simulink model "lab61"  (R2023b)
settings: Solver=VariableStepAuto  StartTime=0.0  StopTime=100  RelTol=1e-3
model workspace (MAT data in the model file):
  a = 0.12271788776
  u = 6.36307057012e-06
libraries: checkpacklib x1
settings Model: Creator=Настя  LastModifiedBy=killer
settings SolverCC: AlgebraicLoopSolver=TrustRegion
settings DebuggingCC: UnconnectedInputMsg=warning  UnconnectedOutputMsg=warning  UnconnectedLineMsg=warning
settings ModelReferenceCC: EnableRefExpFcnMdlSchedulingChecks=on
settings RTWCC: DLArmComputeVersion=19.05

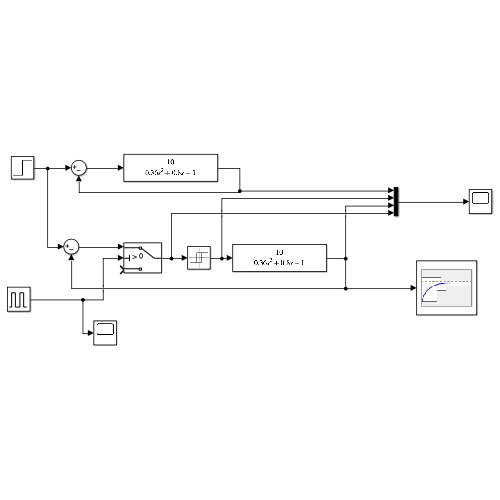
[thumbnail: Simulink's stored preview of the top-level diagram]
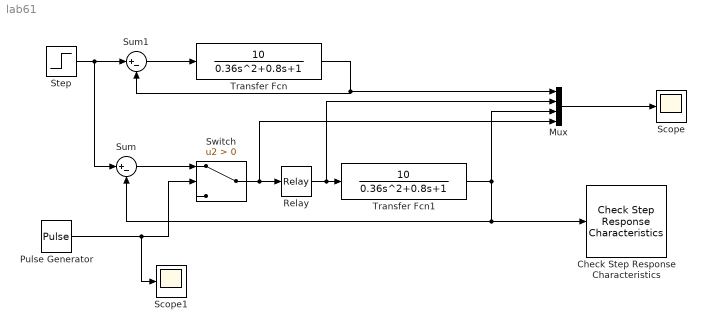
== system lab61 ==
  Check Step Response Characteristics : checkpacklib/Check Step Response  Characteristics  InstantiateOnLoad=on  enabled=on  stopWhenAssertionFail=off  export=off  ViewDlgPos=[]  OpenViewOnLoad=off  LaunchViewOnOpen=off  TimeUnits=seconds  EnableStepResponseBound=on  InitialValue=0  FinalValue=1  StepTime=0  RiseTime=5  PercentRise=80  SettlingTime=7  PercentSettling=1  PercentOvershoot=10  PercentUndershoot=1
  Mux : Mux
  Pulse Generator : DiscretePulseGenerator  PulseType=Time based  Period=0.008  PulseWidth=50
  Relay : Relay  OnSwitchValue=u  OffSwitchValue=-u  OnOutputValue=a  OffOutputValue=-a
  Scope : Scope
  Scope1 : Scope
  Step : Step  Time=0  SampleTime=0
  Sum : Sum  Inputs=|+-
  Sum1 : Sum  Inputs=|+-
  Switch : Switch  Criteria=u2 > Threshold  SaturateOnIntegerOverflow=off  InputSameDT=off
  Transfer Fcn : TransferFcn  Numerator=[10]  Denominator=[0.36 0.8 1]
  Transfer Fcn1 : TransferFcn  Numerator=[10]  Denominator=[0.36 0.8 1]
  wires:
  Sum1/1 -> Transfer Fcn/1
  Transfer Fcn/1 -> Sum1/2, Mux/1
  Relay/1 -> Transfer Fcn1/1, Mux/2
  Mux/1 -> Scope/1
  Transfer Fcn1/1 -> Sum/2, Check Step Response Characteristics/1, Mux/3
  Switch/1 -> Mux/4, Relay/1
  Step/1 -> Sum/1, Sum1/1
  Sum/1 -> Switch/1
  Pulse Generator/1 -> Scope1/1, Switch/2
